simulink model "simulation_"  (R2021a)
settings: Solver=ode1  StartTime=0.0  StopTime=30  FixedStep=1e-5  RelTol=1e-3
values from neighbouring files (symbols this model uses):
  tc = 1    [before_simulation.m]    (also in elasticity.m)
  v0 = 10    [before_simulation.m]
settings Model: Creator=Buyson  LastModifiedBy=Buyson

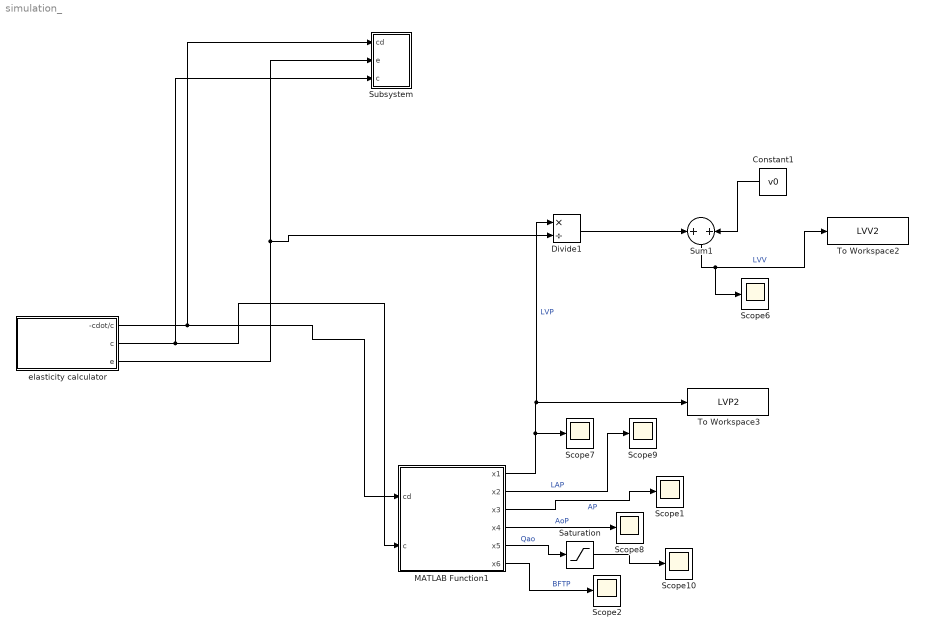
== system simulation_ ==
  Constant1 : Constant  Value=v0
  Divide1 : Product  Inputs=*/
  MATLAB Function1 : MATLAB Function  TreatAsAtomicUnit=on
  Saturation : Saturate  UpperLimit=770  LowerLimit=0
  Scope{1..2,6..10} (7 alike) : Scope
  Subsystem : Subsystem
  Sum1 : Sum  Inputs=+|+
  To Workspace2 : ToWorkspace  VariableName=LVV2  SampleTime=-1
  To Workspace3 : ToWorkspace  VariableName=LVP2  SampleTime=-1
  elasticity calculator : Subsystem
  wires:
  elasticity calculator/1(-cdot/c) -> Subsystem/1(cd), MATLAB Function1/1(cd)
  elasticity calculator/2(c) -> MATLAB Function1/2(c), Subsystem/3(c)
  MATLAB Function1/2(x2) -> Scope9/1  "LAP"
  MATLAB Function1/3(x3) -> Scope1/1  "AP"
  MATLAB Function1/4(x4) -> Scope8/1  "AoP"
  MATLAB Function1/6(x6) -> Scope2/1  "BFTP"
  Divide1/1 -> Sum1/1
  Constant1/1 -> Sum1/2
  Sum1/1 -> Scope6/1, To Workspace2/1  "LVV"
  elasticity calculator/3(e) -> Divide1/2, Subsystem/2(e)
  MATLAB Function1/1(x1) -> Divide1/1, To Workspace3/1, Scope7/1  "LVP"
  MATLAB Function1/5(x5) -> Saturation/1  "Qao"
  Saturation/1 -> Scope10/1

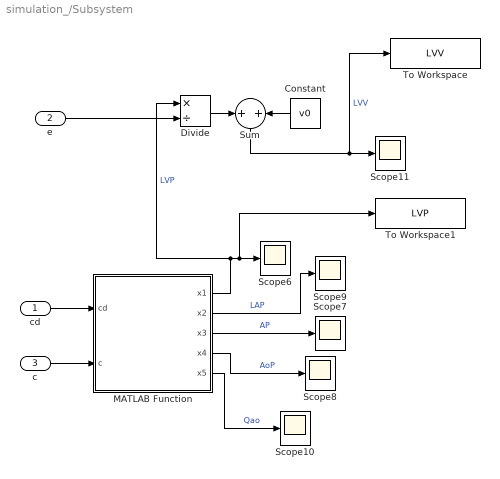
== system simulation_/Subsystem ==
  cd : Inport
  e : Inport  Port=2
  c : Inport  Port=3
  Constant : Constant  Value=v0
  Divide : Product  Inputs=*/
  MATLAB Function : MATLAB Function  TreatAsAtomicUnit=on
  Scope{6..11} (6 alike) : Scope
  Sum : Sum  Inputs=+|+
  To Workspace : ToWorkspace  VariableName=LVV  SampleTime=-1
  To Workspace1 : ToWorkspace  VariableName=LVP  SampleTime=-1
  wires:
  MATLAB Function/5(x5) -> Scope10/1  "Qao"
  MATLAB Function/1(x1) -> Scope6/1, To Workspace1/1, Divide/1  "LVP"
  e/1 -> Divide/2
  MATLAB Function/4(x4) -> Scope8/1  "AoP"
  MATLAB Function/3(x3) -> Scope7/1  "AP"
  MATLAB Function/2(x2) -> Scope9/1  "LAP"
  Sum/1 -> Scope11/1, To Workspace/1  "LVV"
  Constant/1 -> Sum/2
  Divide/1 -> Sum/1
  cd/1 -> MATLAB Function/1(cd)
  c/1 -> MATLAB Function/2(c)

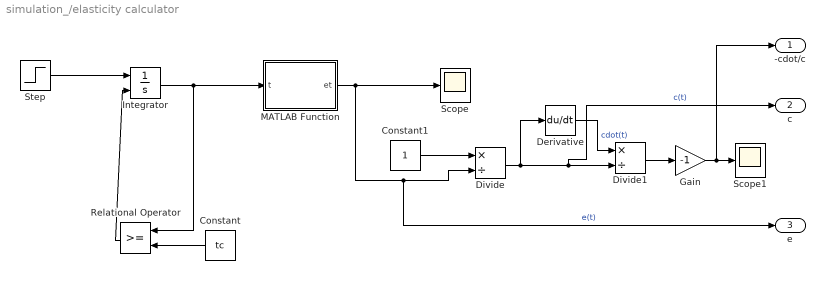
== system simulation_/elasticity calculator ==
  Constant : Constant  Value=tc
  Constant1 : Constant
  Derivative : Derivative
  Divide : Product  Inputs=*/
  Divide1 : Product  Inputs=*/
  Gain : Gain  Gain=-1
  Integrator : Integrator  ExternalReset=rising
  MATLAB Function : MATLAB Function  TreatAsAtomicUnit=on
  Relational Operator : RelationalOperator  OutDataTypeStr=boolean  RndMeth=Simplest
  Scope : Scope
  Scope1 : Scope
  Step : Step  Time=0  SampleTime=0
  -cdot/c : Outport
  c : Outport  Port=2
  e : Outport  Port=3
  wires:
  Divide1/1 -> Gain/1
  Constant/1 -> Relational Operator/2
  Constant1/1 -> Divide/1
  Gain/1 -> Scope1/1, -cdot/c/1
  Step/1 -> Integrator/1
  Relational Operator/1 -> Integrator/2
  MATLAB Function/1(et) -> e/1, Divide/2, Scope/1  "e(t)"
  Integrator/1 -> Relational Operator/1, MATLAB Function/1(t)
  Derivative/1 -> Divide1/1  "cdot(t)"
  Divide/1 -> Derivative/1, c/1, Divide1/2  "c(t)"

== matlab function simulation_/Subsystem/MATLAB Function ==
  settings: updateMethod=DISCRETE
  data: cd input; x1 output; c input; x2 output; x3 output; x4 output; x5 output
function [x1,x2,x3,x4,x5]= fcn(cd, c)
persistent x1up x2up x3up x4up x5up;
% persistent aup;
if (isempty(x1up) || isempty(x2up) || isempty(x3up) || isempty(x4up) || isempty(x5up)) 
    x1up = 8.5; %lvp
    x2up = 7; %lap
    x3up = 75; %ap -->???????????????????
    x4up = 75; %aop
    x5up = 0; %qao
%     x1up = 10;
%     x2up = 10;
%     x3up = 10;
%     x4up = 10;
%     x5up = 10;
%     aup = -1;
end
rs = 1; rm = 0.005; ra = 0.001; rc = 0.0398;
cr = 4.4; cs = 1.33; ca = 0.08; ls = 0.0005;

dt = 1e-5;
x1 = x1up + dt * (cd * x1up + 1/c*(1/rm*fun(x2up - x1up) - 1/ra*fun(x1up - x4up)));
x2 = x2up + dt * (1/(rs*cr)*(x3up - x2up) - 1/(cr*rm)*fun(x2up - x1up));
x3 = x3up + dt * (1/(rs*cs)*(-x3up + x2up) + x5up/cs);
x4 = x4up + dt * (-x5up/ca + 1/(ca*ra)*fun(x1up - x4up));
x5 = x5up + dt * (1/ls*(-x3up + x4up - rc * x5up));
% a = aup + fun(aup);
x1up = x1;
x2up = x2;
x3up = x3;
x4up = x4;
x5up = x5;
% aup = a;
    function val = fun(m)
        if(m >= 0)
            val = m;
        else
            val = 0;
        end
    end

end

== matlab function simulation_/elasticity calculator/MATLAB Function ==
  data: t input; et output
function et = fcn(t)
HR = 60;
tc = 60/HR;
tmax = 0.2+0.15*tc;
tn = t/tmax;
en = 1.55*((tn/0.7)^(1.9)/(1 + (tn/0.7)^(1.9)))*(1/(1 + (tn/1.17)^(21.9)));
emax = 2;emin = 0.06;
et = (emax - emin)*en + emin;

== matlab function simulation_/MATLAB Function1 ==
  settings: updateMethod=DISCRETE
  data: cd input; x1 output; c input; x2 output; x3 output; x4 output; x5 output; x6 output
function [x1,x2,x3,x4,x5,x6]= fcn2(cd, c)
persistent x1up x2up x3up x4up x5up x6up;
if (isempty(x1up) || isempty(x2up) || isempty(x3up) || isempty(x4up) || isempty(x5up) || isempty(x6up)) 
    x1up = 8.5; %lvp
    x2up = 7; %lap
    x3up = 75; %ap -->???????????????????
    x4up = 75; %aop
    x5up = 0; %qao
    x6up = 12; %new state
end
rs = 1; rm = 0.8; ra = 0.001; rc = 0.0398;
cr = 4.4; cs = 1.33; ca = 0.08; ls = 0.0005;
%% new
x1h = 1; alpha = 1;
if(x1up > x1h)
    rk = alpha*(x1up - x1h);
%     rk = 0;
else
%     rk = -alpha*(x1up - x1h);
    rk = 0;
end
ri = 0.0677; ro = 0.0677; li = 0.0127; lo = 0.0127;
b0 = -0.1707; b1 = -0.0218; b2 = 9.9e-07; w = 2000;
las = li + lo + b1; ras = ri + ro + rk + b0;
%%

dt = 1e-5;
x1 = x1up + dt * (cd * x1up + 1/c*(1/rm*fun(x2up - x1up) - 1/ra*fun(x1up - x4up)) -1/c*x6up);
x2 = x2up + dt * (1/(rs*cr)*(x3up - x2up) - 1/(cr*rm)*fun(x2up - x1up));
x3 = x3up + dt * (1/(rs*cs)*(-x3up + x2up) + x5up/cs);
x4 = x4up + dt * (-x5up/ca + 1/(ca*ra)*fun(x1up - x4up) + x6up/ca);
x5 = x5up + dt * (1/ls*(-x3up + x4up - rc * x5up));
x6 = x6up + dt * (1/las*(x1up - x4up - ras * x6up)) - b2/las * w^2;

x1up = x1;
x2up = x2;
x3up = x3;
x4up = x4;
x5up = x5;
x6up = x6;
    function val = fun(m)
        if(m >= 0)
            val = m;
        else
            val = 0;
        end
    end

end
